simulink library "INT_InjCtl_qCoSync"  (R2016b)
settings: Solver=VariableStepAuto  StartTime=0.0  StopTime=10.0  RelTol=1e-3
settings Model: Creator=zhoutinglin  LastModifiedBy=zhoutinglin

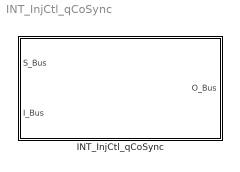
== system INT_InjCtl_qCoSync ==
  INT_InjCtl_qCoSync : Subsystem

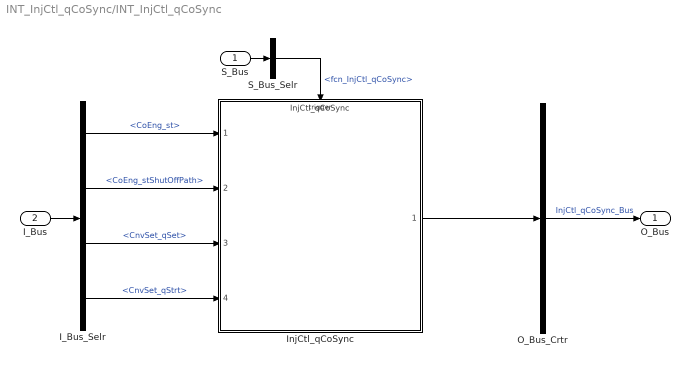
== system INT_InjCtl_qCoSync/INT_InjCtl_qCoSync ==
  S_Bus : Inport
  I_Bus : Inport  Port=2
  I_Bus_Selr : BusSelector  OutputSignals=CoEng_st,CoEng_stShutOffPath,CnvSet_qSet,CnvSet_qStrt
  InjCtl_qCoSync : ModelReference  ModelNameDialog=InjCtl_qCoSync  SimulationMode=Normal  ModelReferenceVersion=1.7  TriggerPortName=function  TriggerPortTriggerType=function-call  TriggerPortStatesWhenEnabling=held
  O_Bus_Crtr : BusCreator  Inputs=1
  S_Bus_Selr : BusSelector  OutputSignals=fcn_InjCtl_qCoSync
  O_Bus : Outport
  wires:
  S_Bus_Selr/1 -> InjCtl_qCoSync/Trigger  "<fcn_InjCtl_qCoSync>"
  S_Bus/1 -> S_Bus_Selr/1
  I_Bus/1 -> I_Bus_Selr/1
  I_Bus_Selr/1 -> InjCtl_qCoSync/1  "<CoEng_st>"
  I_Bus_Selr/2 -> InjCtl_qCoSync/2  "<CoEng_stShutOffPath>"
  I_Bus_Selr/3 -> InjCtl_qCoSync/3  "<CnvSet_qSet>"
  I_Bus_Selr/4 -> InjCtl_qCoSync/4  "<CnvSet_qStrt>"
  O_Bus_Crtr/1 -> O_Bus/1  "InjCtl_qCoSync_Bus"
  InjCtl_qCoSync/1 -> O_Bus_Crtr/1
